simulink model "mitrule_normalize"  (R2022b)
settings: Solver=VariableStepAuto  StartTime=0.0  StopTime=300  RelTol=1e-3
values from neighbouring files (symbols this model uses):
  den = [1 2*zeta*omega omega^2]    [parameter.m]
  L_deltaa = ((rho*s*v^2*b)/2*I_xx)*c_ldeltaa    (= 0.0088445952)    [parameter.m]
  L_p = ((rho*s*v*b^2)/4*I_xx)*c_lp    (= -0.007578712512)    [parameter.m]
  num = [omega^2]    [parameter.m]
libraries: matrix_library x2
settings Model: Creator=110  LastModifiedBy=110

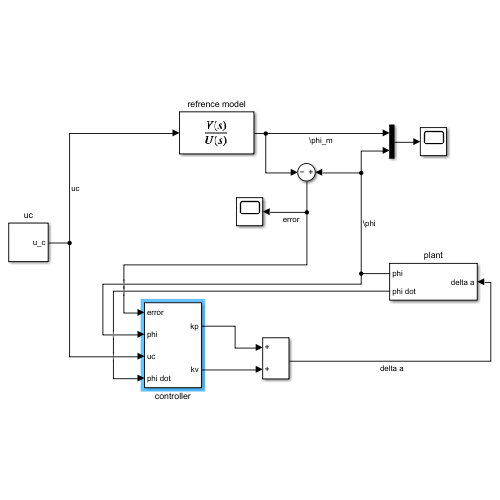
[thumbnail: Simulink's stored preview of the top-level diagram]
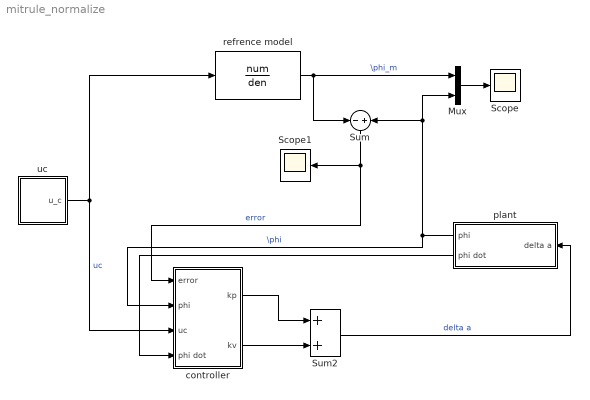
== system mitrule_normalize ==
  Mux : Mux  Inputs=2
  Scope : Scope
  Scope1 : Scope
  Sum : Sum  Inputs=-+
  Sum2 : Sum
  controller : Subsystem
  plant : Subsystem
  refrence model : TransferFcn  Numerator=num  Denominator=den
  uc : Subsystem
  wires:
  plant/1(phi) -> Sum/2, Mux/2, controller/2(phi)  "\\phi"
  plant/2(phi dot) -> controller/4(phi dot)
  Sum2/1 -> plant/1(delta a)  "delta a"
  Sum/1 -> controller/1(error), Scope1/1  "error"
  controller/2(kv) -> Sum2/2
  controller/1(kp) -> Sum2/1
  refrence model/1 -> Mux/1, Sum/1  "\\phi_m"
  uc/1(u_c) -> controller/3(uc), refrence model/1  "uc"
  Mux/1 -> Scope/1

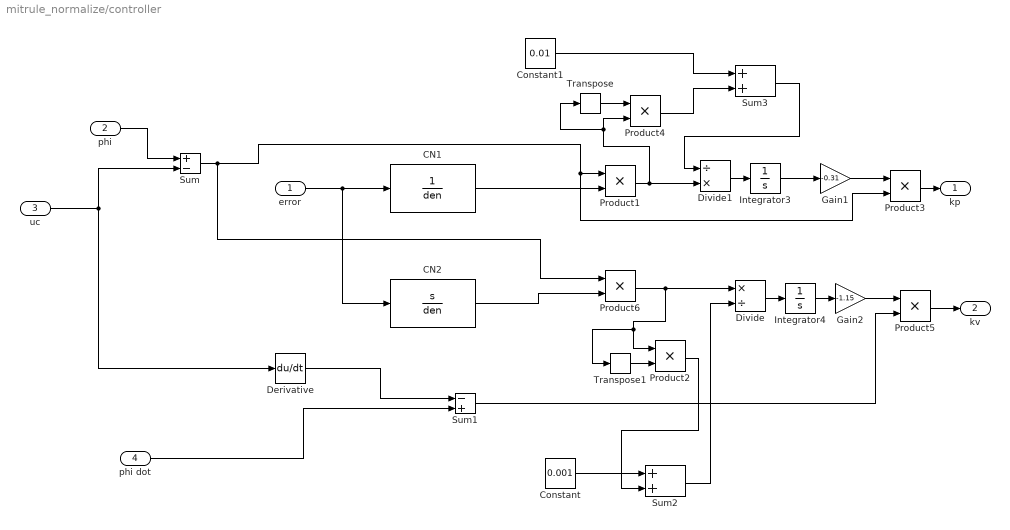
== system mitrule_normalize/controller ==
  error : Inport
  phi : Inport  Port=2
  uc : Inport  Port=3
  phi dot : Inport  Port=4
  CN1 : TransferFcn  Numerator=1  Denominator=den
  CN2 : TransferFcn  Numerator=[1 0]  Denominator=den
  Constant : Constant  Value=0.001
  Constant1 : Constant  Value=0.01
  Derivative : Derivative
  Divide : Product  Inputs=*/
  Divide1 : Product  Inputs=/*
  Gain1 : Gain  Gain=-0.31
  Gain2 : Gain  Gain=-1.15
  Integrator3 : Integrator
  Integrator4 : Integrator
  Product{1..6} (6 alike) : Product
  Sum : Sum  Inputs=+-
  Sum1 : Sum  Inputs=-+
  Sum2 : Sum
  Sum3 : Sum
  Transpose : matrix_library/Transpose
  Transpose1 : matrix_library/Transpose
  kp : Outport
  kv : Outport  Port=2
  wires:
  Gain2/1 -> Product5/1
  Integrator4/1 -> Gain2/1
  Integrator3/1 -> Gain1/1
  Gain1/1 -> Product3/1
  Product5/1 -> kv/1
  Product3/1 -> kp/1
  phi/1 -> Sum/1
  uc/1 -> Derivative/1, Sum/2
  Sum/1 -> Product6/1, Product1/1, Product3/2
  error/1 -> CN2/1, CN1/1
  CN2/1 -> Product6/2
  CN1/1 -> Product1/2
  phi dot/1 -> Sum1/2
  Derivative/1 -> Sum1/1
  Sum1/1 -> Product5/2
  Constant/1 -> Sum2/1
  Product6/1 -> Product2/1, Transpose1/1, Divide/1
  Product2/1 -> Sum2/2
  Sum2/1 -> Divide/2
  Divide/1 -> Integrator4/1
  Product4/1 -> Sum3/2
  Constant1/1 -> Sum3/1
  Sum3/1 -> Divide1/1
  Product1/1 -> Transpose/1, Product4/2, Divide1/2
  Divide1/1 -> Integrator3/1
  Transpose/1 -> Product4/1
  Transpose1/1 -> Product2/2

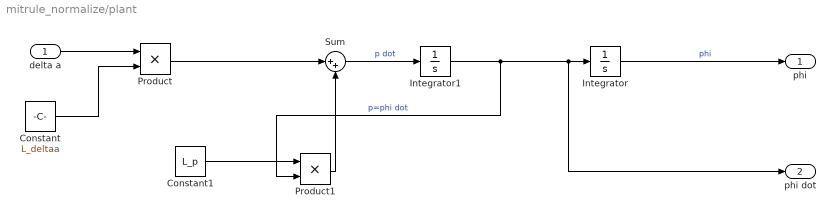
== system mitrule_normalize/plant ==
  delta a : Inport
  Constant : Constant  Value=L_deltaa
  Constant1 : Constant  Value=L_p
  Integrator : Integrator
  Integrator1 : Integrator
  Product : Product
  Product1 : Product
  Sum : Sum  Inputs=|++
  phi : Outport
  phi dot : Outport  Port=2
  wires:
  Integrator/1 -> phi/1  "phi"
  delta a/1 -> Product/1
  Constant/1 -> Product/2
  Product/1 -> Sum/1
  Product1/1 -> Sum/2
  Constant1/1 -> Product1/1
  Sum/1 -> Integrator1/1  "p dot"
  Integrator1/1 -> Product1/2, phi dot/1, Integrator/1  "p=phi dot"

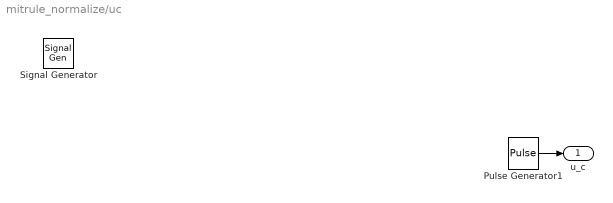
== system mitrule_normalize/uc ==
  Pulse Generator1 : DiscretePulseGenerator  PulseType=Time based  Amplitude=5  Period=20  PulseWidth=50
  Signal Generator : SignalGenerator  WaveForm=square  Amplitude=5  Units=rad/sec
  u_c : Outport
  wires:
  Pulse Generator1/1 -> u_c/1
